simulink model "upPos_bezkompenzace"  (R2016b)
settings: Solver=FixedStepAuto  StartTime=0.0  StopTime=20  FixedStep=prms.Ts  RelTol=1e-3
PreLoadFcn:
  | Ts = 1e-3
undefined symbols (not defined in the file): DiscIntNeverNeededParam, K, P0, prms, x0
libraries: raspi_library x2, simulink x1
PreSaveFcn:
  | set_param(gcs, 'location', [15 50 815 560])
settings Model: SimulationMode=external  Creator=The MathWorks Inc.  LastModifiedBy=gurtnmar
settings SolverCC: PositivePriorityOrder=on
settings DataIOCC: LimitDataPoints=on  SaveFormat=Array
settings OptimizationCC: BlockReduction=off  BooleanDataType=off  DefaultUnderspecifiedDataType=single  LifeSpan=inf  MaxStackSize=64
settings DebuggingCC: SaveWithParameterizedLinksMsg=none  UnderspecifiedInitializationDetection=Classic  MergeDetectMultiDrivingBlocksExec=none  SignalResolutionControl=TryResolveAllWithWarning  ParameterTunabilityLossMsg=error  SFUnexpectedBacktrackingDiag=warning  SFNoUnconditionalDefaultTransitionDiag=warning  SFExecutionAtInitializationDiag=none
settings HardwareCC: ProdBitPerPointer=32  ProdBitPerSizeT=32  ProdBitPerPtrDiffT=32  ProdLargestAtomicInteger=Long  ProdLargestAtomicFloat=Double  ProdWordSize=32  ProdHWDeviceType=ARM Compatible->ARM Cortex
settings ModelReferenceCC: PropagateSignalLabelsOutOfModel=off
settings RTWCC: SystemTargetFile=ert.tlc  HardwareBoard=Raspberry Pi  TLCOptions=-aInlineSetEventsForThisBaseRateFcn=TLC_FALSE -aSuppressMultiTaskScheduler=TLC_FALSE -aRateBasedStepFcn=0  TemplateMakefile=ert_default_tmf  Description=Embedded Coder  GenerateReport=on  RTWVerbose=off  Toolchain=GNU GCC Raspberry Pi  BuildConfiguration=Specify  IncludeHyperlinkInReport=on  GenerateTraceInfo=on  GenerateTraceReport=on  GenerateTraceReportSl=on  GenerateTraceReportSf=on  GenerateTraceReportEml=on
settings CodeAppCC: ForceParamTrailComments=on  IgnoreCustomStorageClasses=off  OperatorAnnotations=on  SimulinkDataObjDesc=on  SFDataObjDesc=on  MATLABFcnDesc=on  MangleLength=10  InsertBlockDesc=on  MATLABSourceComments=on
settings ERTTargetCC: SupportVariableSizeSignals=on
settings ConfigComp: CovMetricSettings=dw  CovHtmlReporting=on  CovSaveCumulativeToWorkspaceVar=on  CovSaveSingleToWorkspaceVar=on  CovExternalEMLEnable=off  CovSFcnEnable=off

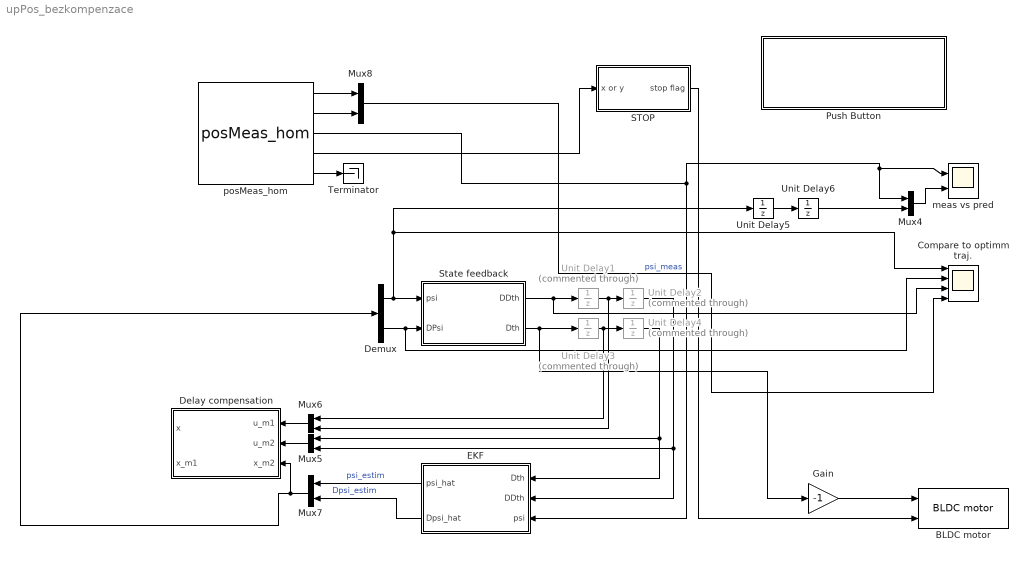
== system upPos_bezkompenzace ==
  BLDC motor : raspi_library/BLDC motor
  Compare to optimm traj. : Scope  NumInputPorts=4
  Delay compensation : Subsystem
  Demux : Demux  Outputs=2
  EKF : Subsystem
  Gain : Gain  Gain=-1
  Mux{4..8} (5 alike) : Mux  Inputs=2
  Push Button : Subsystem  DialogController=hmiCreateDDGDialog  IsWebBlock=on  mask(MWDashboardBlock){webBlockId=aa30e358-d2c6-466c-a89a-de069679829e, webBlockType=pushbutton, ShowInLibBrwoser=on, ShowInitialText=on, HMISrcModelName=upPos_bezkompenzace}
      mask prompts: webBlockId "WebBlock Id"; webBlockType "WebBlock Type"; HMISrcModelName "Source Model"
      mask help: SimulinkHMI:dialogs:PushButtonDialogDesc
      mask Help: helpview([docroot '/mapfiles/simulink.map'], 'hmi_push_button')
      mask Display:
      | model = bdroot(gcb);
      | if strcmp(get_param(model,'BlockDiagramType'), 'library')
      |     image([(matlabroot) '/toolbox/simulink/hmi/icons/PushButton.png']);
      | end
  STOP : Subsystem
  State feedback : Subsystem
  Terminator : Terminator
  Unit Delay{1..4} (4 alike) : UnitDelay  Commented=through  SampleTime=-1
  Unit Delay5 : UnitDelay  SampleTime=-1
  Unit Delay6 : UnitDelay  SampleTime=-1
  meas vs pred : Scope  NumInputPorts=2
  posMeas_hom : raspi_library/posMeas_hom
  wires:
  posMeas_hom/3 -> meas vs pred/1, Mux4/1, EKF/3(psi)  "psi_meas"
  Demux/1 -> State feedback/1(psi), Compare to optimm traj./1, Unit Delay5/1
  Unit Delay1/1 -> Mux6/2, Unit Delay2/1
  Mux5/1 -> Delay compensation/2(u_m2)
  Mux6/1 -> Delay compensation/1(u_m1)
  EKF/2(Dpsi_hat) -> Mux7/2  "Dpsi_estim"
  EKF/1(psi_hat) -> Mux7/1  "psi_estim"
  Unit Delay2/1 -> EKF/2(DDth), Mux5/2
  Unit Delay4/1 -> Mux5/1, EKF/1(Dth)
  Unit Delay3/1 -> Mux6/1, Unit Delay4/1
  Mux7/1 -> Delay compensation/3(x_m2), Demux/1
  Demux/2 -> Compare to optimm traj./2, State feedback/2(DPsi)
  State feedback/1(DDth) -> Compare to optimm traj./3, Unit Delay1/1
  STOP/1(stop flag) -> BLDC motor/2
  Mux4/1 -> meas vs pred/2
  Unit Delay6/1 -> Mux4/2
  Unit Delay5/1 -> Unit Delay6/1
  posMeas_hom/5 -> Terminator/1
  posMeas_hom/4 -> STOP/1(x or y)
  posMeas_hom/1 -> Mux8/1
  posMeas_hom/2 -> Mux8/2
  Mux8/1 -> Compare to optimm traj./4
  State feedback/2(Dth) -> Gain/1, Unit Delay3/1
  Gain/1 -> BLDC motor/1

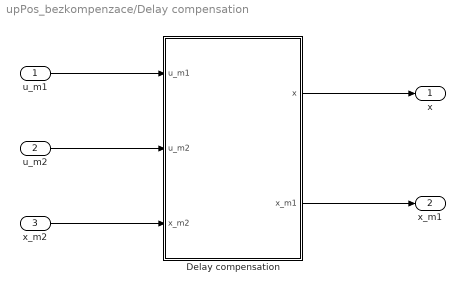
== system upPos_bezkompenzace/Delay compensation ==
  u_m1 : Inport
  u_m2 : Inport  Port=2
  x_m2 : Inport  Port=3
  Delay compensation : MATLAB Function  TreatAsAtomicUnit=on  SystemSampleTime=prms.Ts
  x : Outport
  x_m1 : Outport  Port=2
  wires:
  x_m2/1 -> Delay compensation/3(x_m2)
  u_m1/1 -> Delay compensation/1(u_m1)
  u_m2/1 -> Delay compensation/2(u_m2)
  Delay compensation/1(x) -> x/1
  Delay compensation/2(x_m1) -> x_m1/1

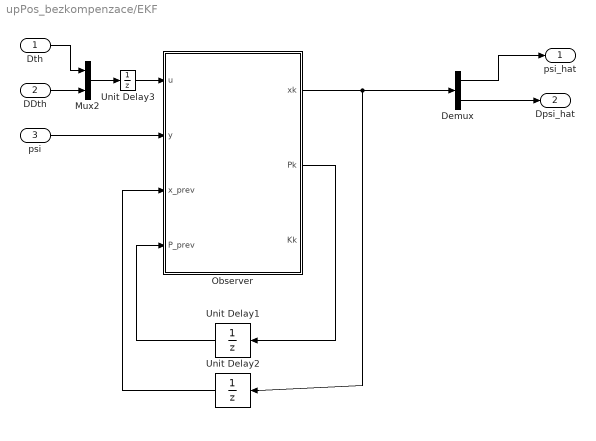
== system upPos_bezkompenzace/EKF ==
  Dth : Inport
  DDth : Inport  Port=2
  psi : Inport  Port=3
  Demux : Demux  Outputs=2
  Mux2 : Mux  Inputs=2
  Observer : MATLAB Function  TreatAsAtomicUnit=on  SystemSampleTime=prms.Ts
  Unit Delay1 : UnitDelay  InitialCondition=P0  SampleTime=-1
  Unit Delay2 : UnitDelay  InitialCondition=x0  SampleTime=-1
  Unit Delay3 : UnitDelay  SampleTime=-1
  psi_hat : Outport
  Dpsi_hat : Outport  Port=2
  wires:
  Unit Delay2/1 -> Observer/3(x_prev)
  Observer/2(Pk) -> Unit Delay1/1
  Unit Delay1/1 -> Observer/4(P_prev)
  Observer/1(xk) -> Demux/1, Unit Delay2/1
  Demux/2 -> Dpsi_hat/1
  Demux/1 -> psi_hat/1
  Mux2/1 -> Unit Delay3/1
  Dth/1 -> Mux2/1
  DDth/1 -> Mux2/2
  psi/1 -> Observer/2(y)
  Unit Delay3/1 -> Observer/1(u)

== system upPos_bezkompenzace/Push Button ==

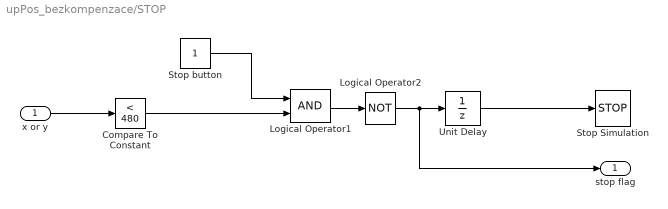
== system upPos_bezkompenzace/STOP ==
  x or y : Inport
  Compare To Constant : simulink/Logic and Bit Operations/Compare To Constant  relop=<  const=480  OutDataTypeStr=boolean
  Logical Operator1 : Logic  AllPortsSameDT=off  OutDataTypeStr=boolean
  Logical Operator2 : Logic  Operator=NOT  AllPortsSameDT=off  OutDataTypeStr=boolean
  Stop Simulation : Stop
  Stop button : Constant
  Unit Delay : UnitDelay  SampleTime=-1
  stop flag : Outport
  wires:
  Unit Delay/1 -> Stop Simulation/1
  Logical Operator2/1 -> stop flag/1, Unit Delay/1
  Compare To Constant/1 -> Logical Operator1/2
  Stop button/1 -> Logical Operator1/1
  x or y/1 -> Compare To Constant/1
  Logical Operator1/1 -> Logical Operator2/1

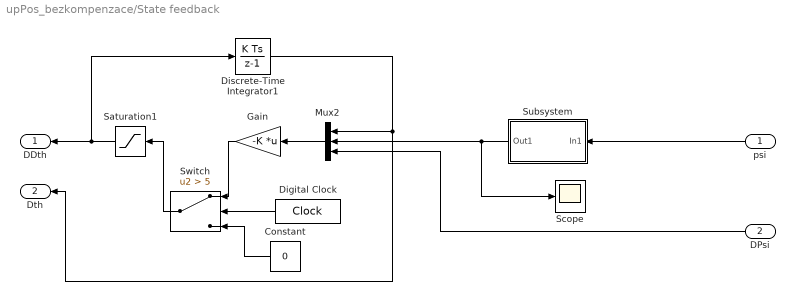
== system upPos_bezkompenzace/State feedback ==
  psi : Inport
  DPsi : Inport  Port=2
  Constant : Constant  Value=0  OutDataTypeStr=single
  Digital Clock : DigitalClock  SampleTime=prms.Ts
  Discrete-Time Integrator1 : DiscreteIntegrator  InitialConditionSetting=State (most efficient)  SampleTime=prms.Ts  LimitOutput=on  UpperSaturationLimit=38  LowerSaturationLimit=-38  ICPrevOutput=DiscIntNeverNeededParam  ICPrevScaledInput=DiscIntNeverNeededParam
  Gain : Gain  Gain=-K  Multiplication=Matrix(K*u)
  Mux2 : Mux  Inputs=3
  Saturation1 : Saturate  UpperLimit=prms.usat  LowerLimit=-prms.usat
  Scope : Scope
  Subsystem : Subsystem
  Switch : Switch  Criteria=u2 > Threshold  Threshold=5
  DDth : Outport
  Dth : Outport  Port=2
  wires:
  Saturation1/1 -> Discrete-Time Integrator1/1, DDth/1
  Discrete-Time Integrator1/1 -> Dth/1, Mux2/1
  DPsi/1 -> Mux2/3
  Mux2/1 -> Gain/1
  Subsystem/1(Out1) -> Scope/1, Mux2/2
  psi/1 -> Subsystem/1(In1)
  Switch/1 -> Saturation1/1
  Gain/1 -> Switch/1
  Constant/1 -> Switch/3
  Digital Clock/1 -> Switch/2

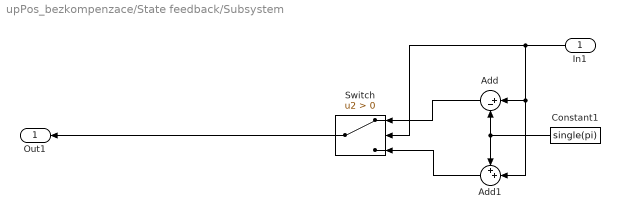
== system upPos_bezkompenzace/State feedback/Subsystem ==
  In1 : Inport
  Add : Sum  Inputs=|+-
  Add1 : Sum  Inputs=++|
  Constant1 : Constant  Value=single(pi)
  Switch : Switch  Criteria=u2 > Threshold
  Out1 : Outport
  wires:
  Add/1 -> Switch/1
  Switch/1 -> Out1/1
  Add1/1 -> Switch/3
  Constant1/1 -> Add/2, Add1/1
  In1/1 -> Add1/2, Add/1, Switch/2

== matlab function upPos_bezkompenzace/Delay compensation/Delay compensation ==
  data: u_m1 input; u_m2 input; x output; x_m2 input; prms parameter; x_m1 output
function [x, x_m1] = delayCompensation( u_m1, u_m2, x_m2, prms)

a =  prms.out.a_bar;
b =  prms.out.b_bar;
c =  prms.out.c_bar;
d =  prms.out.d_bar;
e =  prms.out.e_bar;

N = 1;
T = prms.Ts/N;

% Time Update - 1
x_old = x_m2;
x_new = single([0; 0]);
for i = 1:N
    x_new(1) = x_old(1) + T*x_old(2);
    x_new(2) = x_old(2) + T* 1/a*(-c*sin(x_old(1)) - b*x_old(2) - d*u_m2(1) + e*u_m2(2));    
    x_old = x_new;
end
x_m1 = x_new;

% Time Update - 2
x_old = x_m1;
x_new = single([0; 0]);
for i = 1:N
    x_new(1) = x_old(1) + T*x_old(2);
    x_new(2) = x_old(2) + T*1/a*(-c*sin(x_old(1)) - b*x_old(2) - d*u_m1(1) + e*u_m1(2));    
    x_old = x_new;
end
x = x_new;

== matlab function upPos_bezkompenzace/EKF/Observer ==
  data: u input; y input; xk output single; x_prev input; P_prev input; Pk output; Kk output; prms parameter
function [xk, Pk, Kk] = EKF( u, y, x_prev, P_prev, prms)

a =  prms.out.a_bar;
b =  prms.out.b_bar;
c =  prms.out.c_bar;
d =  prms.out.d_bar;
e =  prms.out.e_bar;

Q =  prms.out.KF.Q;
R =  prms.out.KF.R;

Ak_c = [0 1; -c/a*cos(x_prev(1)) -b/a]; % system matrix of the linearized continuous model
Ak = eye(2) + prms.Ts*Ak_c; % discretized version of the system matrix
Hk = [1 0];

% Time Update
xk = single([0; 0]);
xk(1) = x_prev(1) + prms.Ts*x_prev(2);
xk(2) = x_prev(2) + prms.Ts * 1/a*(-c*sin(x_prev(1)) - b*x_prev(2) - d*u(1) + e*u(2));
% xk = Ak*x_prev + Bk*u;
Pk = Ak*P_prev*Ak'+Q;

% Measurement Update
Kk = Pk*Hk'/(Hk*Pk*Hk'+R);
xk = xk + Kk*(y-Hk*xk);
Pk = (eye(2)-Kk*Hk)*Pk;
